simulink model "stream_fft"  (R2021a)
settings: Solver=VariableStepAuto  StartTime=0.0  StopTime=0  RelTol=1e-3
undefined symbols (not defined in the file): S, vsva2197, xcvc1902
libraries: aieBasic x4, dspsrcs4 x2, aieUtilities x2, dspxfrm3 x1, aieDSP x1, vmcUtilities x1
settings Model: Creator=ravidapu  LastModifiedBy=abehbood
settings SolverCC: AlgebraicLoopSolver=TrustRegion

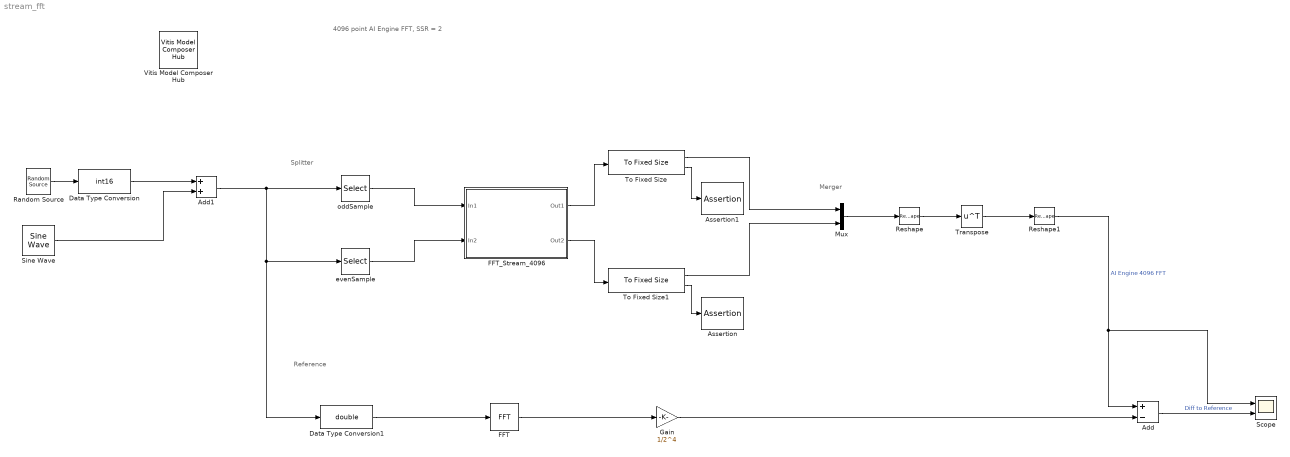
== system stream_fft ==
  note: Reference
  note: Splitter
  note: Merger
  note: 4096 point AI Engine FFT, SSR = 2
  Add : Sum  Inputs=+-  OutDataTypeStr=double
  Add1 : Sum
  Assertion : Assertion
  Assertion1 : Assertion
  Data Type Conversion : DataTypeConversion  OutDataTypeStr=int16
  Data Type Conversion1 : DataTypeConversion  OutDataTypeStr=double
  FFT : dspxfrm3/FFT  FFTImplementation=Auto  CompMethod=Table lookup  TableOpt=NEW  TableOptActive=Speed  BitRevOrder=off  Normalize=off  InheritFFTLength=on  FFTLength=64  WrapInput=on  roundingMode=Floor  overflowMode=off  firstCoeffDataTypeStr=Inherit: Same word length as input  firstCoeffLastDataTypeStr=Inherit: Same word length as input  outputMin=[]  outputMax=[]
  FFT_Stream_4096 : Subsystem
  Gain : Gain  Gain=1/2^4
  Mux : Mux  Inputs=2
  Random Source : dspsrcs4/Random Source  SrcType=Uniform  NormMethod=Ziggurat  CltLength=12  MinVal=-5  MaxVal=5  MeanVal=0  VarVal=1  RepMode=Not repeatable  rawSeed=1  IsInherit=off  SampMode=Discrete  SampTime=1  SampFrame=4096  DataType=Double  OutComplex=Complex  OutputFrames=off
  Reshape : Reshape  OutputDimensionality=Customize  OutputDimensions=[4096/2, 2]
  Reshape1 : Reshape  OutputDimensions=[1, 10]
  Scope : Scope  NumInputPorts=2
  Sine Wave : dspsrcs4/Sine Wave  Amplitude=50  Frequency=1/10  Phase=0  SampleMode=Discrete  OutComplex=Real  CompMethod=Table lookup  TableSize=Speed  SampleTime=1  SamplesPerFrame=4096  ResetState=Restart at time zero  OutputFrames=off  dataType=Fixed-point  wordLen=16  udDataType=sfix(16)  fracBitsMode=User-defined  numFracBits=0  OutDataTypeStr=fixdt(1,16,0)  LastOutDataTypeStr=fixdt(1,16,0)
  To Fixed Size : aieUtilities/To Fixed Size  OutputSize=Inherit: Same as input  CopyMethod=Buffer samples to form output  HasStatusOutput=off
  To Fixed Size1 : aieUtilities/To Fixed Size  OutputSize=Inherit: Same as input  CopyMethod=Buffer samples to form output  HasStatusOutput=off
  Transpose : Math  Operator=transpose  SaturateOnIntegerOverflow=on
  Vitis Model Composer Hub : vmcUtilities/Vitis Model Composer Hub  Tag=genX  CodeGeneration=off  SubsystemName=DUT  TargetDirectory=./code  ExportType=AI Engines  IpVendor=xilinx.com  IpLibrary=hls  IpVersion=1.0  IpHWLanguage=Verilog  AieCompilerOptions={}  CreateTestbench=off  TestbenchStackSize=10  RunAieSim=off  AieSimTimeout=50000  RunAieSimProfiling=off  LaunchVitisAnalyzer=off  PlotOutput=off  RunX86Sim=off  X86SimTimeout=10  GenHwImage=off  PlatformType=Not Specified  HwSystemType=Baremetal  HwValidationTarget=hw  ProjDevice=xcvc1902-vsva2197-2MP-e-S  ProjDevicePart=xcvc1902-vsva2197-2MP-e-S  SamplePeriod=-1  ClockFrequency=200  DataPathParallelism=1  xilinxfamily=Kintex7  part=xc7k325t  speed=-3  package=fbg676  directory=./netlist  testbench=off  incr_netlist=off  synthesis_tool=Vivado  clock_wrapper=Clock Enables  dbl_ovrd=According to Block Masks  dcm_input_clock_period=10  sysclk_period=10  simulink_period=1  eval_field=0
  evenSample : Selector  InputPortWidth=4096  IndexOptions=Index vector (dialog)  Indices=2:2:4096  OutputSizes=1
  oddSample : Selector  InputPortWidth=4096  IndexOptions=Index vector (dialog)  Indices=1:2:4096  OutputSizes=1
  wires:
  evenSample/1 -> FFT_Stream_4096/2(In2)
  oddSample/1 -> FFT_Stream_4096/1(In1)
  FFT_Stream_4096/1(Out1) -> To Fixed Size/1
  FFT_Stream_4096/2(Out2) -> To Fixed Size1/1
  Reshape1/1 -> Add/1, Scope/1  "AI Engine 4096 FFT"
  FFT/1 -> Gain/1
  To Fixed Size/1 -> Mux/1
  Transpose/1 -> Reshape1/1
  Reshape/1 -> Transpose/1
  Mux/1 -> Reshape/1
  To Fixed Size1/1 -> Mux/2
  Add/1 -> Scope/2  "Diff to Reference"
  Data Type Conversion/1 -> Add1/1
  Add1/1 -> oddSample/1, evenSample/1, Data Type Conversion1/1
  Sine Wave/1 -> Add1/2
  Random Source/1 -> Data Type Conversion/1
  Data Type Conversion1/1 -> FFT/1
  To Fixed Size1/2 -> Assertion/1
  To Fixed Size/2 -> Assertion1/1
  Gain/1 -> Add/2

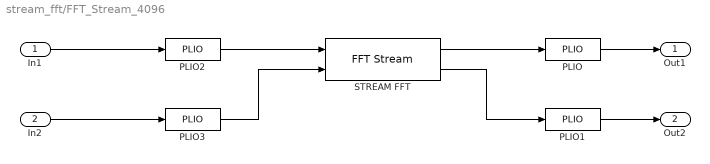
== system stream_fft/FFT_Stream_4096 ==
  In1 : Inport
  In2 : Inport  Port=2
  PLIO{,1..3} (4 alike) : aieBasic/PLIO  PlioWidth=64  PlioFreqSpec=off  PlioFreq=250  ColLocation=0  channel=0  blockJsonConstraints=[]  deprecateConstraints=0
  STREAM FFT : aieDSP/FFT Stream  data_type=cint16  point_size=4096  input_window_size=4096  shift_val=4  ssr=2  input_sampling_rate=200  use_casc_length=on  casc_length=1  spec=meta_data_hl_stream_fft.json
  Out1 : Outport
  Out2 : Outport  Port=2
  wires:
  In1/1 -> PLIO2/1
  STREAM FFT/2 -> PLIO1/1
  STREAM FFT/1 -> PLIO/1
  In2/1 -> PLIO3/1
  PLIO/1 -> Out1/1
  PLIO1/1 -> Out2/1
  PLIO2/1 -> STREAM FFT/1
  PLIO3/1 -> STREAM FFT/2
